simulink model "PI_sim"  (R2021b)
settings: Solver=VariableStepAuto  StartTime=0.0  StopTime=100.0  RelTol=1e-3
undefined symbols (not defined in the file): Ki, Kp, pGain, pT, upb
settings Model: Creator=Ondrej  LastModifiedBy=Administrator

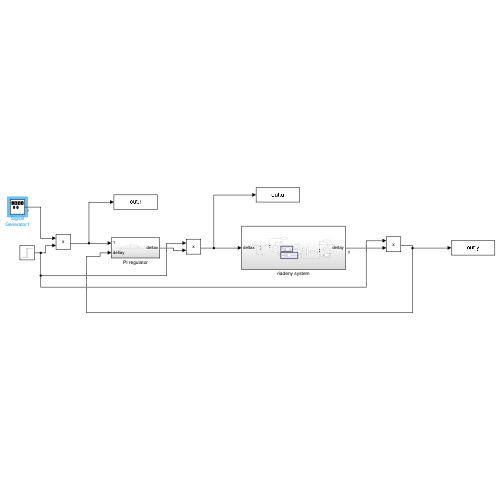
[thumbnail: Simulink's stored preview of the top-level diagram]
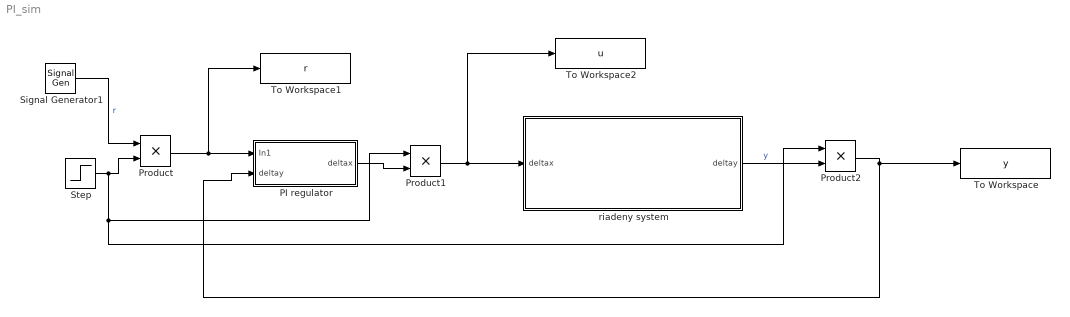
== system PI_sim ==
  PI regulator : Subsystem
  Product : Product
  Product1 : Product
  Product2 : Product
  Signal Generator1 : SignalGenerator  WaveForm=square  Amplitude=-2  Frequency=1/10
  Step : Step  Time=2  SampleTime=0
  To Workspace : ToWorkspace  VariableName=y  SaveFormat=Timeseries  SampleTime=-1
  To Workspace1 : ToWorkspace  VariableName=r  SaveFormat=Timeseries  SampleTime=-1
  To Workspace2 : ToWorkspace  VariableName=u  SaveFormat=Timeseries  SampleTime=-1
  riadeny system : Subsystem
  wires:
  Signal Generator1/1 -> Product/1  "r"
  Step/1 -> Product2/1, Product1/1, Product/2
  Product/1 -> PI regulator/1(In1), To Workspace1/1
  PI regulator/1(deltax) -> Product1/2
  Product1/1 -> To Workspace2/1, riadeny system/1(deltax)
  riadeny system/1(deltay) -> Product2/2  "y"
  Product2/1 -> To Workspace/1, PI regulator/2(deltay)

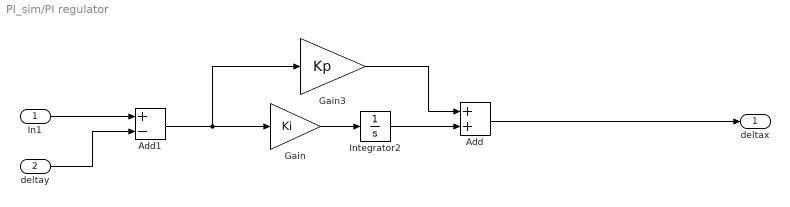
== system PI_sim/PI regulator ==
  In1 : Inport
  deltay : Inport  Port=2
  Add : Sum
  Add1 : Sum  Inputs=+-
  Gain : Gain  Gain=Ki
  Gain3 : Gain  Gain=Kp
  Integrator2 : Integrator
  deltax : Outport
  wires:
  Integrator2/1 -> Add/2
  Add/1 -> deltax/1
  Gain/1 -> Integrator2/1
  Gain3/1 -> Add/1
  Add1/1 -> Gain3/1, Gain/1
  In1/1 -> Add1/1
  deltay/1 -> Add1/2

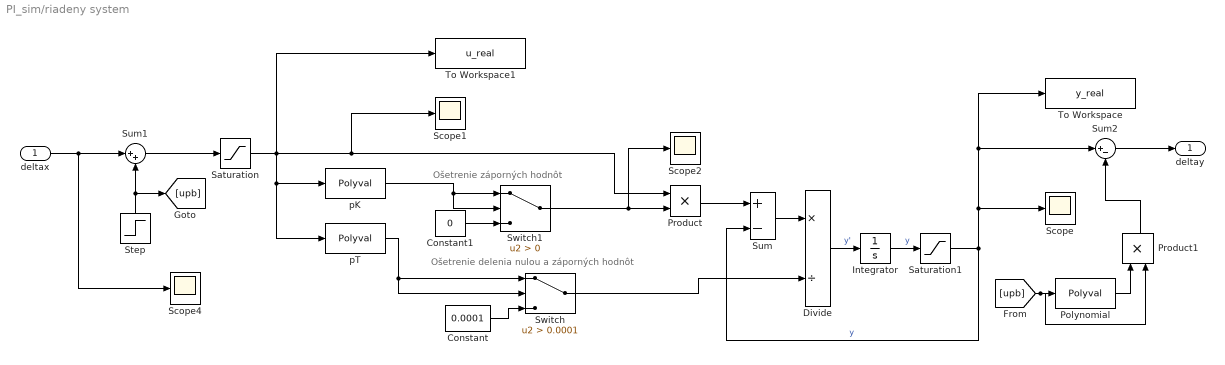
== system PI_sim/riadeny system ==
  note: Ošetrenie delenia nulou a záporných hodnôt
  note: Ošetrenie záporných hodnôt
  deltax : Inport
  Constant : Constant  Value=0.0001
  Constant1 : Constant  Value=0
  Divide : Product  Inputs=*/
  Integrator : Integrator
  Polynomial : Polyval  Coefs=pGain
  Product : Product
  Product1 : Product
  Saturation : Saturate  UpperLimit=255  LowerLimit=0
  Saturation1 : Saturate  UpperLimit=1023  LowerLimit=0
  Scope{,1..2,4} (4 alike) : Scope
  Step : Step  Time=50  Before=upb  After=upb-upb_delta  SampleTime=0
  Sum : Sum  Inputs=+-
  Sum1 : Sum  Inputs=|++
  Sum2 : Sum  Inputs=|+-
  Switch : Switch  Criteria=u2 > Threshold  Threshold=0.0001
  Switch1 : Switch  Criteria=u2 > Threshold
  To Workspace : ToWorkspace  VariableName=y_real  SaveFormat=Timeseries  SampleTime=-1
  To Workspace1 : ToWorkspace  VariableName=u_real  SaveFormat=Timeseries  SampleTime=-1
  pK : Polyval  Coefs=pGain
  pT : Polyval  Coefs=pT
  deltay : Outport
  wires:
  Sum/1 -> Divide/1
  Saturation1/1 -> To Workspace/1, Sum2/1, Scope/1, Sum/2  "y"
  Constant/1 -> Switch/3
  pT/1 -> Switch/1, Switch/2
  pK/1 -> Switch1/2, Switch1/1
  Switch/1 -> Divide/2
  Constant1/1 -> Switch1/3
  Product/1 -> Sum/1
  Switch1/1 -> Scope2/1, Product/2
  Integrator/1 -> Saturation1/1  "y"
  Divide/1 -> Integrator/1  "y'"
  deltax/1 -> Scope4/1, Sum1/1
  Sum1/1 -> Saturation/1
  Saturation/1 -> To Workspace1/1, pT/1, pK/1, Scope1/1, Product/1
  Sum2/1 -> deltay/1
  Polynomial/1 -> Product1/1
  Step/1 -> [upb], Sum1/2
  [upb] -> Product1/2, Polynomial/1
  Product1/1 -> Sum2/2
